simulink library "LumAerospaceBlockset_FlightParameters"  (R2018b)
settings: Solver=ode45  StartTime=0.0  StopTime=10.0  RelTol=1e-3  EnableMultiTasking=on
undefined symbols (not defined in the file): magnitude
libraries: aerolibasang x2, $bdroot x1
settings Model: Creator=Christopher  LastModifiedBy=Christopher
settings DataIOCC: LimitDataPoints=on  SaveFormat=Array
settings OptimizationCC: LifeSpan=inf
settings DebuggingCC: SolverPrmCheckMsg=warning  SFUnexpectedBacktrackingDiag=warning  SFNoUnconditionalDefaultTransitionDiag=warning  SFExecutionAtInitializationDiag=none
settings HardwareCC: ProdBitPerPointer=32  ProdBitPerSizeT=32  ProdBitPerPtrDiffT=32  ProdLargestAtomicFloat=None  ProdIntDivRoundTo=Undefined  ProdEndianess=Unspecified  ProdWordSize=32  ProdHWDeviceType=32-bit Generic
settings ModelReferenceCC: PropagateSignalLabelsOutOfModel=off
settings SFSimCC: SimUseLocalCustomCode=off
settings RTWCC: RTWUseLocalCustomCode=off
settings CodeAppCC: StateflowObjectComments=on
settings GRTTargetCC: TargetLangStandard=C89/C90 (ANSI)  GeneratePreprocessorConditionals=Disable all
settings ConfigComp: CovMetricSettings=dw  CovHtmlReporting=on  CovSaveCumulativeToWorkspaceVar=on  CovSaveSingleToWorkspaceVar=on  CovExternalEMLEnable=off  CovSFcnEnable=off

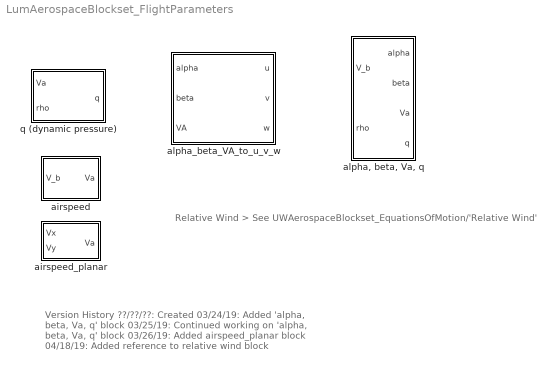
== system LumAerospaceBlockset_FlightParameters ==
  note: Version History
      | ??/??/??: Created
      | 03/24/19: Added 'alpha, beta, Va, q' block
      | 03/25/19: Continued working on 'alpha, beta, Va, q' block
      | 03/26/19: Added airspeed_planar block
      | 04/18/19: Added reference to relative wind block
  note: Relative Wind > See UWAerospaceBlockset_EquationsOfMotion/'Relative Wind'
  airspeed : Subsystem
      mask help:
      | Compute the airspeed from the velocity vector using Va = ||V_b||.
      |
      | INPUT:
      | -V_b: 3x1 vector of velocity
      |
      | OUTPUT:
      | -Va: scalar of the airspeed
      |
      | Created by Christopher Lum
      | lum@uw.edu
  airspeed_planar : Subsystem
      mask help:
      | Calculates the planar airsppeed.
      |
      | INPUTS
      | -Vx: X comopoent of velocity
      | -Vy: Y component of velocity
      |
      | OUTPUTS
      | -Va: Scalar of the airspeed.
      |
      | Created by Christopher Lum
      | lum@uw.edu
  "alpha, beta, Va, q" : Subsystem
      mask help:
      | This block combines the 'Incidence, Sideslip, & Airspeed' and the 'Dynamic Pressure' block from the Aerospace Blockset.
      |
      | In addition, this takes into account the situation where u, v, w are all zero and outputs zero values instead of NaN values.  This makes it more appropriate for situations such as a multi-rotor which has the ability to obtain zero velocity.
      |
      | INPUT:
      | -V_b: 3x1 vector of velocity (m/s)
      | -rho: air density (kg/m^3)
      |
      | OUTPUT:
      | -alpha: angle of attack (rad)
      | -beta: angle of sideslip (rad)
      | -Va: airspeed (m/s)
      | -q: dynamic pressure (N/m^2)
      |
      | Created by Christopher Lum
      | lum@uw.edu
  alpha_beta_VA_to_u_v_w : Subsystem
      mask help:
      | Convert alpha, beta, and VA, to equivalent body velocities, u, v, and, w using
      |
      |     u = VA*cos(alpha)*cos(beta)
      |     v = VA*sin(beta)
      |     w = VA*sin(alpha)cos(beta)
      |
      | INPUT:
      | -alpha:  angle of attack (rad)
      | -beta:   angle of sideslip (rad)
      | -VA:     airspeed (m/s)
      |
      | OUTPUT:
      | -u:      body x velocity (m/s)
      | -v:      body y velocity (m/s)
      | -w:      body z velocity (m/s)
      |
      | Created by Christopher Lum
      | lum@uw.edu
  q (dynamic pressure) : Subsystem
      mask help:
      | Compute dynamic pressure as
      |
      |     q = 0.5*rho*Va^2
      |
      | INPUT:
      | -Va:     airspeed (m/s)
      | -rho:    density (kg/m^3)
      |
      | OUTPUT:
      | -q:      dynamic pressure (N/m^2)
      |
      | See Mathworks Aerospace Blockset, 'Dynamic Pressure' block for a version that accepts a 3x1 vector for the input velocity.
      |
      | Created by Christopher Lum
      | lum@uw.edu

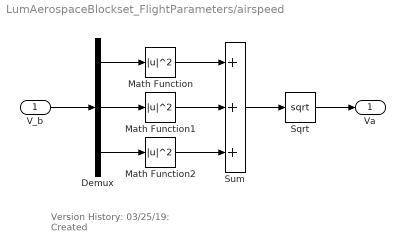
== system LumAerospaceBlockset_FlightParameters/airspeed ==
  note: Version History:
      | 03/25/19: Created
  V_b : Inport
  Demux : Demux  Outputs=3
  Math Function : Math  Operator=magnitude^2  SaturateOnIntegerOverflow=on
  Math Function1 : Math  Operator=magnitude^2  SaturateOnIntegerOverflow=on
  Math Function2 : Math  Operator=magnitude^2  SaturateOnIntegerOverflow=on
  Sqrt : Sqrt  SaturateOnIntegerOverflow=on
  Sum : Sum  Inputs=+++
  Va : Outport
  wires:
  V_b/1 -> Demux/1
  Demux/1 -> Math Function/1
  Demux/2 -> Math Function1/1
  Demux/3 -> Math Function2/1
  Math Function/1 -> Sum/1
  Math Function1/1 -> Sum/2
  Math Function2/1 -> Sum/3
  Sum/1 -> Sqrt/1
  Sqrt/1 -> Va/1

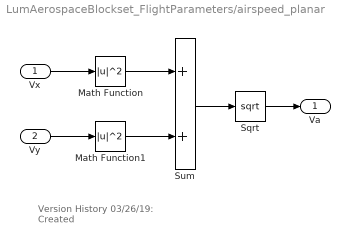
== system LumAerospaceBlockset_FlightParameters/airspeed_planar ==
  note: Version History
      | 03/26/19: Created
  Vx : Inport
  Vy : Inport  Port=2
  Math Function : Math  Operator=magnitude^2  SaturateOnIntegerOverflow=on
  Math Function1 : Math  Operator=magnitude^2  SaturateOnIntegerOverflow=on
  Sqrt : Sqrt  SaturateOnIntegerOverflow=on
  Sum : Sum
  Va : Outport
  wires:
  Math Function/1 -> Sum/1
  Sum/1 -> Sqrt/1
  Sqrt/1 -> Va/1
  Vx/1 -> Math Function/1
  Math Function1/1 -> Sum/2
  Vy/1 -> Math Function1/1

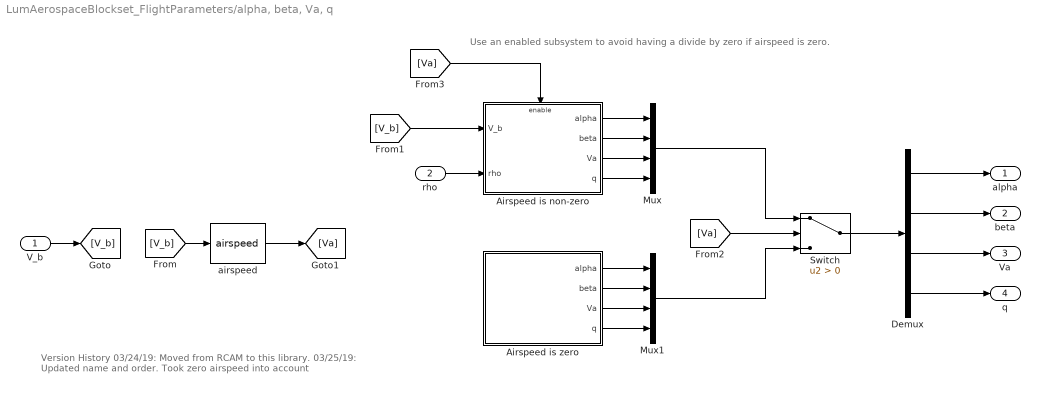
== system LumAerospaceBlockset_FlightParameters/alpha, beta, Va, q ==
  note: Use an enabled subsystem to avoid having a divide by zero if airspeed is zero.
  note: Version History
      | 03/24/19: Moved from RCAM to this library.
      | 03/25/19: Updated name and order.  Took zero airspeed into account
  V_b : Inport
  rho : Inport  Port=2
  "Airspeed is non-zero " : Subsystem
  Airspeed is zero : Subsystem
  Demux : Demux
  Mux : Mux
  Mux1 : Mux
  Switch : Switch  Criteria=u2 > Threshold
  airspeed : $bdroot/airspeed
  alpha : Outport
  beta : Outport  Port=2
  Va : Outport  Port=3
  q : Outport  Port=4
  wires:
  V_b/1 -> [V_b]
  [V_b] -> airspeed/1
  rho/1 -> "Airspeed is non-zero "/2(rho)
  [V_b] -> "Airspeed is non-zero "/1(V_b)
  airspeed/1 -> [Va]
  [Va] -> Switch/2
  "Airspeed is non-zero "/1(alpha) -> Mux/1
  "Airspeed is non-zero "/2(beta) -> Mux/2
  "Airspeed is non-zero "/3(Va) -> Mux/3
  "Airspeed is non-zero "/4(q) -> Mux/4
  Airspeed is zero/1(alpha) -> Mux1/1
  Airspeed is zero/2(beta) -> Mux1/2
  Airspeed is zero/3(Va) -> Mux1/3
  Airspeed is zero/4(q) -> Mux1/4
  Mux1/1 -> Switch/3
  Demux/1 -> alpha/1
  Demux/2 -> beta/1
  Demux/3 -> Va/1
  Demux/4 -> q/1
  Mux/1 -> Switch/1
  Switch/1 -> Demux/1
  [Va] -> "Airspeed is non-zero "/Enable

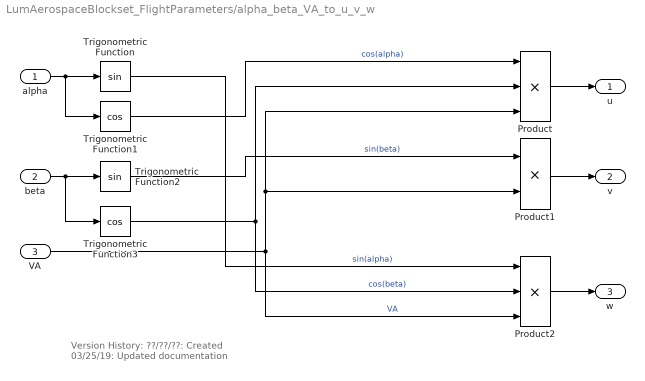
== system LumAerospaceBlockset_FlightParameters/alpha_beta_VA_to_u_v_w ==
  note: Version History:
      | ??/??/??: Created
      | 03/25/19: Updated documentation
  alpha : Inport
  beta : Inport  Port=2
  VA : Inport  Port=3
  Product : Product  Inputs=3  RndMeth=Zero
  Product1 : Product  RndMeth=Zero
  Product2 : Product  Inputs=3  RndMeth=Zero
  Trigonometric Function : Trigonometry
  Trigonometric Function1 : Trigonometry  Operator=cos
  Trigonometric Function2 : Trigonometry
  Trigonometric Function3 : Trigonometry  Operator=cos
  u : Outport
  v : Outport  Port=2
  w : Outport  Port=3
  wires:
  Trigonometric Function/1 -> Product2/1  "sin(alpha)"
  Trigonometric Function2/1 -> Product1/1  "sin(beta)"
  Trigonometric Function1/1 -> Product/1  "cos(alpha)"
  Trigonometric Function3/1 -> Product2/2, Product/2  "cos(beta)"
  Product2/1 -> w/1
  Product1/1 -> v/1
  Product/1 -> u/1
  VA/1 -> Product2/3, Product1/2, Product/3  "VA"
  beta/1 -> Trigonometric Function3/1, Trigonometric Function2/1
  alpha/1 -> Trigonometric Function1/1, Trigonometric Function/1

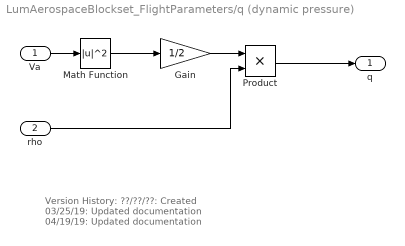
== system LumAerospaceBlockset_FlightParameters/q (dynamic pressure) ==
  note: Version History:
      | ??/??/??: Created
      | 03/25/19: Updated documentation
      | 04/19/19: Updated documentation
  Va : Inport
  rho : Inport  Port=2
  Gain : Gain  Gain=1/2
  Math Function : Math  Operator=magnitude^2  SaturateOnIntegerOverflow=on
  Product : Product  RndMeth=Zero
  q : Outport
  wires:
  Va/1 -> Math Function/1
  Gain/1 -> Product/1
  Math Function/1 -> Gain/1
  Product/1 -> q/1
  rho/1 -> Product/2

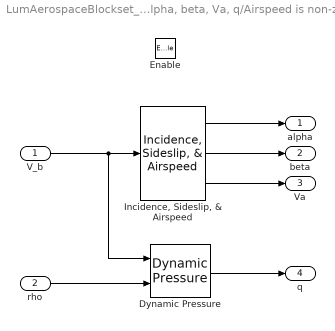
== system LumAerospaceBlockset_FlightParameters/alpha, beta, Va, q/Airspeed is non-zero  ==
  V_b : Inport
  rho : Inport  Port=2
  Enable : EnablePort
  Dynamic Pressure : aerolibasang/Dynamic Pressure
  "Incidence, Sideslip, & Airspeed" : aerolibasang/Incidence, Sideslip, & Airspeed
      settings: SourceProductName=Aerospace Blockset
  alpha : Outport
  beta : Outport  Port=2
  Va : Outport  Port=3
  q : Outport  Port=4
  wires:
  rho/1 -> Dynamic Pressure/2
  V_b/1 -> "Incidence, Sideslip, & Airspeed"/1, Dynamic Pressure/1
  "Incidence, Sideslip, & Airspeed"/1 -> alpha/1
  "Incidence, Sideslip, & Airspeed"/2 -> beta/1
  Dynamic Pressure/1 -> q/1
  "Incidence, Sideslip, & Airspeed"/3 -> Va/1

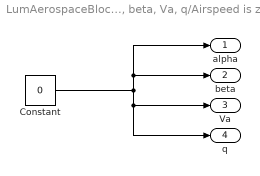
== system LumAerospaceBlockset_FlightParameters/alpha, beta, Va, q/Airspeed is zero ==
  Constant : Constant  Value=0
  alpha : Outport
  beta : Outport  Port=2
  Va : Outport  Port=3
  q : Outport  Port=4
  wires:
  Constant/1 -> alpha/1, beta/1, q/1, Va/1
